simulink model "ModelSim"  (R2025b)
settings: Solver=ode4  StartTime=0.0  StopTime=100  FixedStep=0.005  RelTol=1e-3
undefined symbols (not defined in the file or in its folder): AircraftParam, F, Light, MIL
libraries: aerolibwind2 x3, aerolibsim3d x2, aerolibbdyn x1, sim3dlib x1
settings Model: Creator=pc  LastModifiedBy=pc

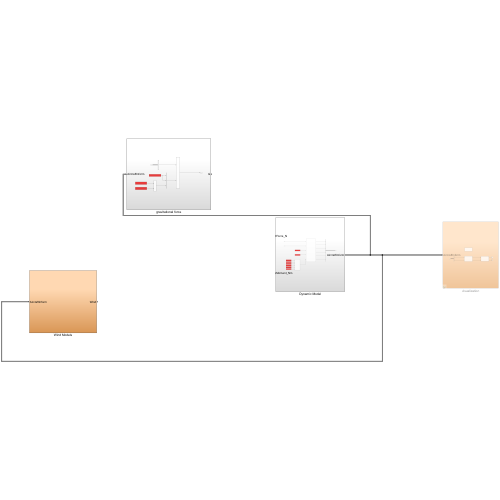
[thumbnail: Simulink's stored preview of the top-level diagram]
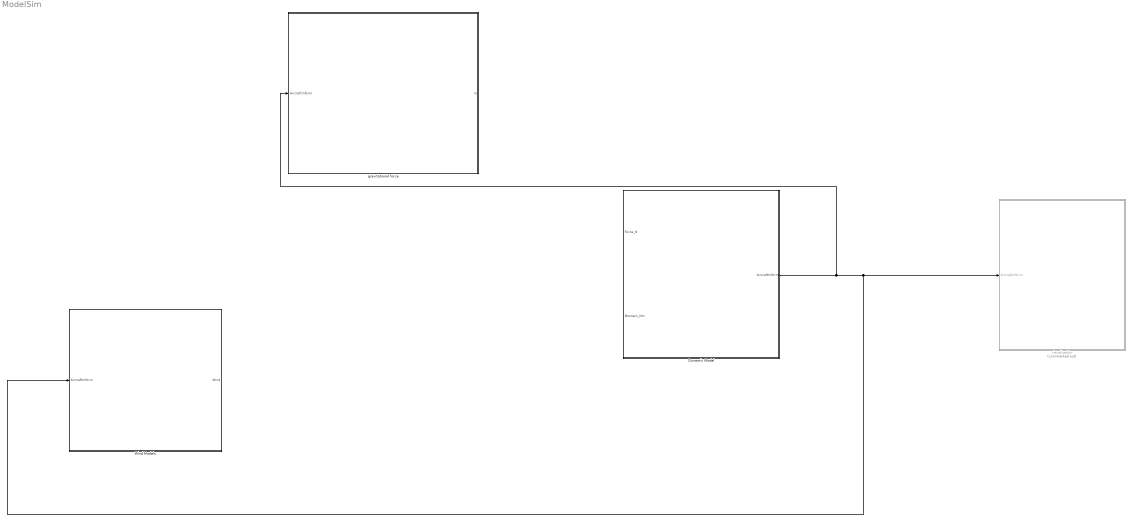
== system ModelSim ==
  Dynamic Model : Subsystem
  Wind Models : Subsystem
  gravitational force : Subsystem
  visualization : Subsystem  Commented=on
  wires:
  Dynamic Model/1(AircraftInform) -> Wind Models/1(AircraftInform), visualization/1(AircraftInform), gravitational force/1(AircraftInform)

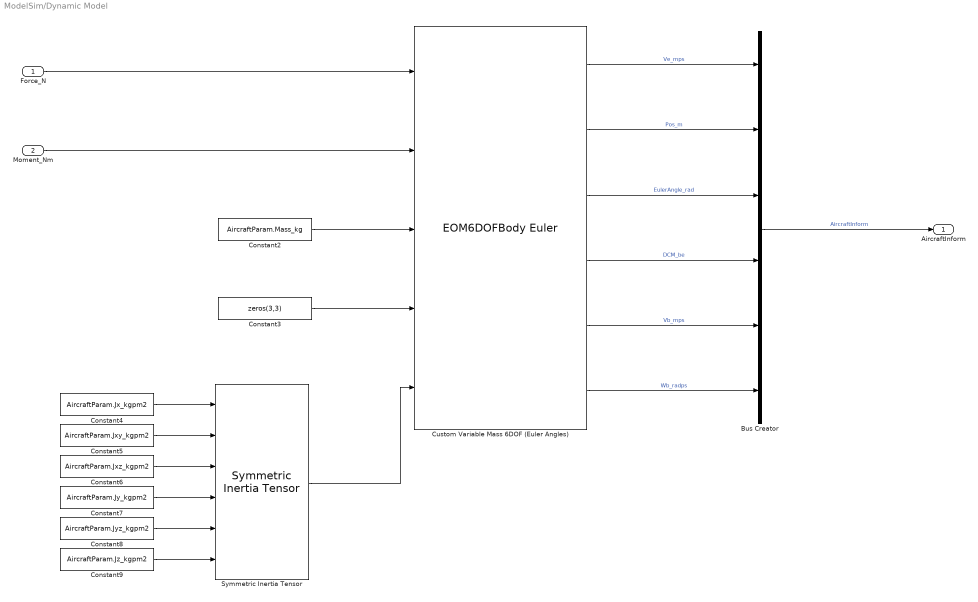
== system ModelSim/Dynamic Model ==
  Force_N : Inport
  Moment_Nm : Inport  Port=2
  Bus Creator : BusCreator  Inputs=6
  Constant2 : Constant  Value=AircraftParam.Mass_kg
  Constant3 : Constant  Value=zeros(3,3)
  Constant4 : Constant  Value=AircraftParam.Jx_kgpm2
  Constant5 : Constant  Value=AircraftParam.Jxy_kgpm2
  Constant6 : Constant  Value=AircraftParam.Jxz_kgpm2
  Constant7 : Constant  Value=AircraftParam.Jy_kgpm2
  Constant8 : Constant  Value=AircraftParam.Jyz_kgpm2
  Constant9 : Constant  Value=AircraftParam.Jz_kgpm2
  Custom Variable Mass 6DOF (Euler Angles) : EOM6DOFBodyEuler  mtype=Custom Variable
  Symmetric Inertia Tensor : aerolibbdyn/Symmetric Inertia Tensor
  AircraftInform : Outport
  wires:
  Custom Variable Mass 6DOF (Euler Angles)/3 -> Bus Creator/3  "EulerAngle_rad"
  Constant6/1 -> Symmetric Inertia Tensor/3
  Constant4/1 -> Symmetric Inertia Tensor/1
  Custom Variable Mass 6DOF (Euler Angles)/2 -> Bus Creator/2  "Pos_m"
  Custom Variable Mass 6DOF (Euler Angles)/4 -> Bus Creator/4  "DCM_be"
  Constant9/1 -> Symmetric Inertia Tensor/6
  Constant7/1 -> Symmetric Inertia Tensor/4
  Custom Variable Mass 6DOF (Euler Angles)/1 -> Bus Creator/1  "Ve_mps"
  Custom Variable Mass 6DOF (Euler Angles)/6 -> Bus Creator/6  "Wb_radps"
  Constant3/1 -> Custom Variable Mass 6DOF (Euler Angles)/4
  Moment_Nm/1 -> Custom Variable Mass 6DOF (Euler Angles)/2
  Custom Variable Mass 6DOF (Euler Angles)/5 -> Bus Creator/5  "Vb_mps"
  Constant8/1 -> Symmetric Inertia Tensor/5
  Constant2/1 -> Custom Variable Mass 6DOF (Euler Angles)/3
  Symmetric Inertia Tensor/1 -> Custom Variable Mass 6DOF (Euler Angles)/5
  Constant5/1 -> Symmetric Inertia Tensor/2
  Force_N/1 -> Custom Variable Mass 6DOF (Euler Angles)/1
  Bus Creator/1 -> AircraftInform/1  "AircraftInform"

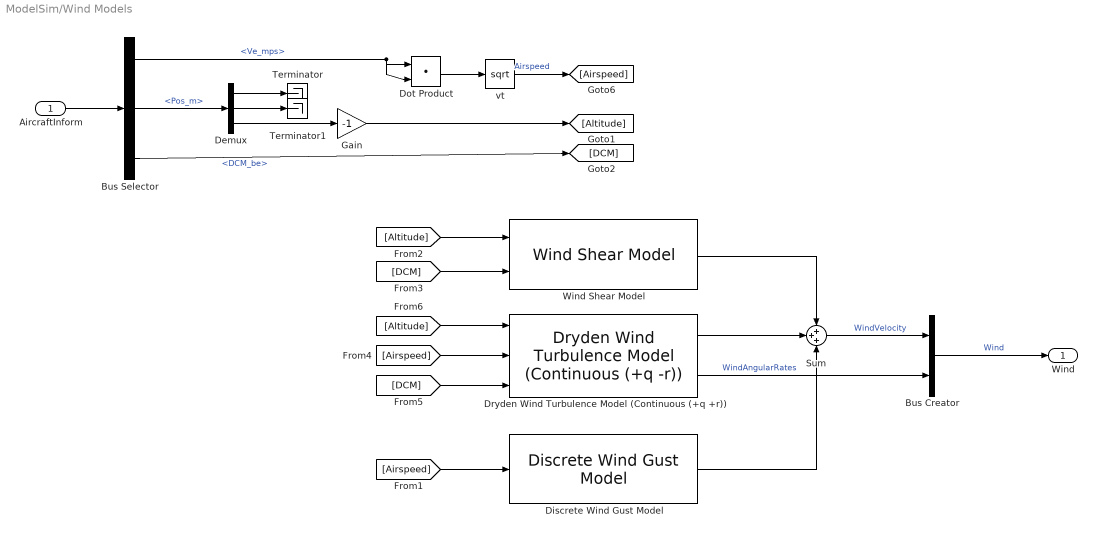
== system ModelSim/Wind Models ==
  AircraftInform : Inport
  Bus Creator : BusCreator  Inputs=2
  Bus Selector : BusSelector  OutputSignals=Ve_mps,Pos_m,DCM_be
  Demux : Demux  Outputs=3
  Discrete Wind Gust Model : aerolibwind2/Discrete Wind Gust Model  units=Metric (MKS)  Gx=off  Gy=off  Gz=off  t_0=20  d_m=[120 120 80]  v_m=[3.5 3.0 3.0]
  Dot Product : DotProduct  InputSameDT=off  OutDataTypeStr=Inherit: Inherit via internal rule
  Dryden Wind Turbulence Model (Continuous (+q +r)) : aerolibwind2/Dryden Wind Turbulence Model  (Continuous (+q -r))  units=Metric (MKS)  spec=MIL-F-8785C  model=Continuous Dryden (+q +r)  W20=5  Wdeg=0  TurbProb=10^-2 - Light  L_high=533.4  Wingspan=AircraftParam.b_m  ts=0.1  Seed=[23341 23342 23343 23344]  T_on=off
  Gain : Gain  Gain=-1
  Sum : Sum  Inputs=+++  InputSameDT=on  SaturateOnIntegerOverflow=on  OutDataTypeStr=Inherit: Same as first input
  Terminator : Terminator
  Terminator1 : Terminator
  Wind Shear Model : aerolibwind2/Wind Shear Model  units=Metric (MKS)  phase=Category C - Terminal Flight Phase  W_20=1  Wdeg=0
  vt : Sqrt
  Wind : Outport
  wires:
  [Altitude] -> Dryden Wind Turbulence Model (Continuous (+q +r))/1
  [DCM] -> Dryden Wind Turbulence Model (Continuous (+q +r))/3
  [DCM] -> Wind Shear Model/2
  Bus Selector/3 -> [DCM]  "<DCM_be>"
  [Altitude] -> Wind Shear Model/1
  Demux/3 -> Gain/1
  [Airspeed] -> Discrete Wind Gust Model/1
  vt/1 -> [Airspeed]  "Airspeed"
  Dot Product/1 -> vt/1
  Dryden Wind Turbulence Model (Continuous (+q +r))/2 -> Bus Creator/2  "WindAngularRates"
  Sum/1 -> Bus Creator/1  "WindVelocity"
  Discrete Wind Gust Model/1 -> Sum/3
  Dryden Wind Turbulence Model (Continuous (+q +r))/1 -> Sum/2
  Wind Shear Model/1 -> Sum/1
  Bus Selector/1 -> Dot Product/2, Dot Product/1  "<Ve_mps>"
  Bus Creator/1 -> Wind/1  "Wind"
  AircraftInform/1 -> Bus Selector/1
  Bus Selector/2 -> Demux/1  "<Pos_m>"
  Gain/1 -> [Altitude]
  Demux/1 -> Terminator/1
  Demux/2 -> Terminator1/1
  [Airspeed] -> Dryden Wind Turbulence Model (Continuous (+q +r))/2

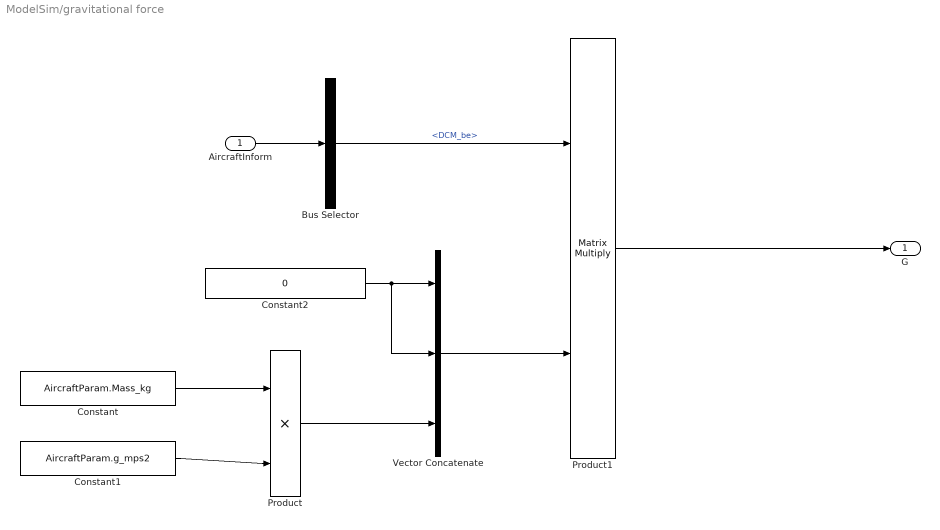
== system ModelSim/gravitational force ==
  AircraftInform : Inport
  Bus Selector : BusSelector  OutputSignals=DCM_be
  Constant : Constant  Value=AircraftParam.Mass_kg
  Constant1 : Constant  Value=AircraftParam.g_mps2
  Constant2 : Constant  Value=0
  Product : Product
  Product1 : Product  Multiplication=Matrix(*)
  Vector Concatenate : Concatenate  NumInputs=3
  G : Outport
  wires:
  Constant/1 -> Product/1
  Constant1/1 -> Product/2
  AircraftInform/1 -> Bus Selector/1
  Bus Selector/1 -> Product1/1  "<DCM_be>"
  Product/1 -> Vector Concatenate/3
  Constant2/1 -> Vector Concatenate/2, Vector Concatenate/1
  Vector Concatenate/1 -> Product1/2
  Product1/1 -> G/1

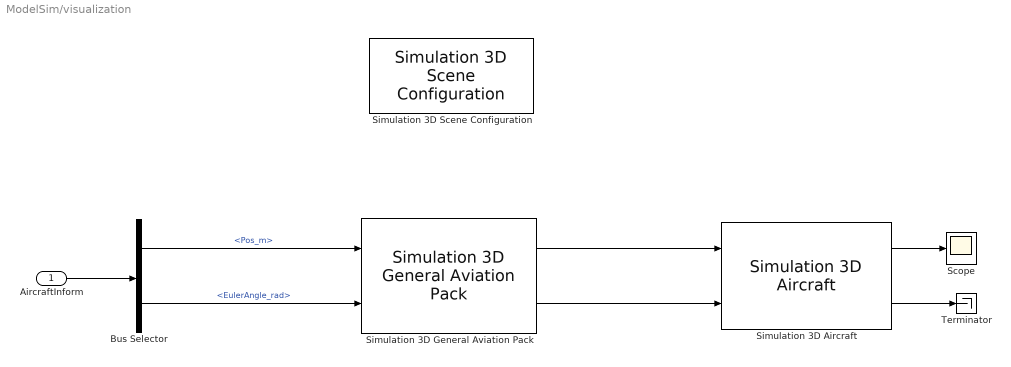
== system ModelSim/visualization ==
  AircraftInform : Inport
  Bus Selector : BusSelector  OutputSignals=Pos_m,EulerAngle_rad
  Scope : Scope
      settings: ActiveDisplayYMinimum=-75.624645429819992  ActiveDisplayYMaximum=411.00234910341749
  Simulation 3D Aircraft : aerolibsim3d/Simulation 3D Aircraft  Priority=-1  Mesh=General aviation  MeshPath=/MathWorksAerospaceContent/Vehicles/Aircraft/Custom/Mesh/SK_HL20.SK_HL20  MeshPathAT=/MathWorksAerospaceContent/Vehicles/Aircraft/AirTransport/Mesh/SK_AirTransport.SK_AirTransport  MeshPathGA=/MathWorksAerospaceContent/Vehicles/Aircraft/GeneralAviation/Mesh/SK_GeneralAviation.SK_GeneralAviation  AircraftColor=Orange  ActorName=SimulinkVehicle1  Translation=zeros( 15, 3 )  Rotation=zeros( 15, 3 )  ScaleInputPort=Dialog  Scale=[1 1 1]  InitialScale=[1 1 1]  IsGHSensorEnabled=on  AreGHRaysVisible=off  IsOutputReshapeEnabled=off  GHRayLength=1524  GHBodyOffset=0.90  GHFrontTireRadius=0.21  GHLeftTireRadius=0.21  GHRightTireRadius=0.21  WoWSensorTolerance=0.05  LightsConfig=Automatic lights  LandingLightIntensity=300000  LandingLightConeAngle=15  CustomLeftLandingLightLocation=[0 0 0]  CustomLeftLandingLightOrientation=[0 0 0]  CustomRightLandingLightLocation=[0 0 0]  CustomRightLandingLightOrientation=[0 0 0]  TaxiLightIntensity=150000  TaxiLightConeAngle=36  CustomTaxiLightLocation=[0 0 0]  CustomTaxiLightOrientation=[0 0 0]  NavLightIntensity=500  PositionLightIntensity=500  StrobeLightIntensity=5000  WingtipStrobePeriod=1.5  WingtipStrobePulseWidth=6  TailStrobePeriod=1.5  TailStrobePulseWidth=6  BeaconLightIntensity=4000  BeaconPeriod=1.5  BeaconPulseWidth=10  SampleTime=-1  ActorType=SimulinkVehicle  ID=1  aMode=0  ActorTag=SimulinkVehicle1
  Simulation 3D General Aviation Pack : aerolibsim3d/Simulation 3D General Aviation Pack  Engine1_T=off  Engine1_R=off  Rudder_T=off  Rudder_R=off  Elevator_T=off  Elevator_R=off  Left_Aileron_T=off  Left_Aileron_R=off  Right_Aileron_T=off  Right_Aileron_R=off  Flaps_T=off  Flaps_R=off  Left_Spoiler_T=off  Left_Spoiler_R=off  Right_Spoiler_T=off  Right_Spoiler_R=off  Nose_Gear_T=off  Nose_Gear_R=off  Nose_Wheel_T=off  Nose_Wheel_R=off  Left_Gear_T=off  Left_Gear_R=off  Left_Wheel_T=off  Left_Wheel_R=off  Right_Gear_T=off  Right_Gear_R=off  Right_Wheel_T=off  Right_Wheel_R=off  EnableUETransform=on  GeoRadioButton=NED
      settings: AttributesFormatString=NED
  Simulation 3D Scene Configuration : sim3dlib/Simulation 3D Scene Configuration  Priority=0  ProjectFormat=Default Scenes  SceneDesc=Airport  ProjectName=D:\MATLAB\toolbox\shared\sim3d_projects\automotive_project_windows\UE\WindowsNoEditor\VehicleSimulation.exe  ScenePath=/Game/Maps/HwStrght  EnableOpenDRIVE=off  vehTagList={'Custom';'Scene Origin';'SimulinkVehicle1'}  vehTag=SimulinkVehicle1  AttachedCameraRelativeTranslation=[0 0 0]  FreeCameraDefaultInitialTranslation=[-6, 0, 2]  AttachedCameraRelativeRotation=[0 0 0]  FreeCameraDefaultInitialRotation=[0, -15, 0]  ViewpointName=Custom  FreeCameraInitialTranslation=[-6, 0, 2]  ViewpointTranslation=[0 0 0]  FreeCameraInitialRotation=[0, -15, 0]  ViewpointRotation=[0 0 0]  OpVisEn=off  Ts=.02  EnableWindow=on  EnableRemoteAccess=off  EnableWeather=off  SunAzimuth=90  SunAltitude=40.0  EnableGeospatialSun=off  Latitude=0  Longitude=0  Date=2023-01-01  Time=10:30:00  GeoTimeZone=-5.0  SunDaylightSaving=off  wind=1  clouds=10  EnableVolumetricClouds=off  CloudCoverage=0  CloudAltitude=6  fog=0  rain=0  RaindropsEffect=off  SnowDensity=0  EnableGeospatial=off  TilesetSource=Earth terrain  UseTrueOrigin=off  OriginHeight=200  OriginLatitude=40.744652  OriginLongitude=-73.988864  MapStyle=Aerial  AdditionalAssetIDs=[]  UseAdvancedSunSky=off  SolarTime=11  TimeZone=-5  Day=21  Month=9  Year=2022  UseDaylightSavingTime=on  DSTStartDay=10  DSTStartMonth=3  DSTEndDay=3  DSTEndMonth=11  DSTSwitchHour=2  sensorTag=MainCamera1  sensorId=1  sensorName=MainCamera1  mountLoc=Origin  offsetFlag=off  tmountOffset=[0, 0, 0]  rmountOffset=[0, 0, 0]  HorizontalResolution=1280  VerticalResolution=720  HorizontalFOV=60  mountPoint=[0 0 0]  mountOrientation=[0 0 0]  aMode=0  ID=1  GeoTrigger=Inactive  ViewNameList={'Custom'}  ViewTranslationList={'[-6 0 2]'}  ViewRotationList={'[0 -15 0]'}
      settings: AttributesFormatString=NED  LibrarySourceBlock=aerolibsim3d/Simulation 3D Scene Configuration
  Terminator : Terminator
  wires:
  Simulation 3D General Aviation Pack/2 -> Simulation 3D Aircraft/2
  Simulation 3D General Aviation Pack/1 -> Simulation 3D Aircraft/1
  Simulation 3D Aircraft/2 -> Terminator/1
  Simulation 3D Aircraft/1 -> Scope/1
  AircraftInform/1 -> Bus Selector/1
  Bus Selector/1 -> Simulation 3D General Aviation Pack/1  "<Pos_m>"
  Bus Selector/2 -> Simulation 3D General Aviation Pack/2  "<EulerAngle_rad>"
